simulink model "sistem_1"  (R2025b)
settings: Solver=VariableStepAuto  StartTime=0.0  StopTime=0.005  RelTol=1e-3
values from neighbouring files (symbols this model uses):
  c = 8e-08    [sistem_1.mat]
  K = 5.9098e-07    [sistem_1.mat]
  k_eq = 0.0291361239712    [sistem_1.mat]
  m_eq = 1.95689925e-12    [sistem_1.mat]
settings Model: Creator=RIZKI  LastModifiedBy=RIZKI

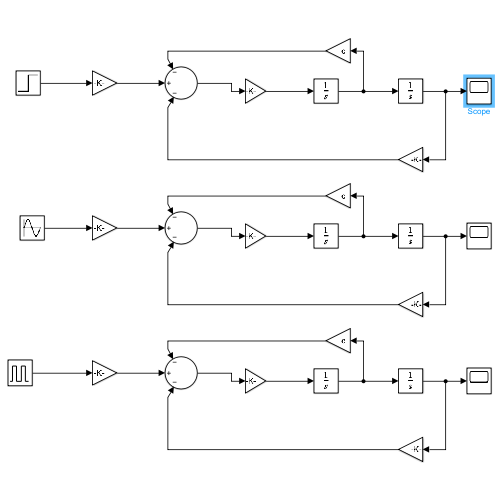
[thumbnail: Simulink's stored preview of the top-level diagram]
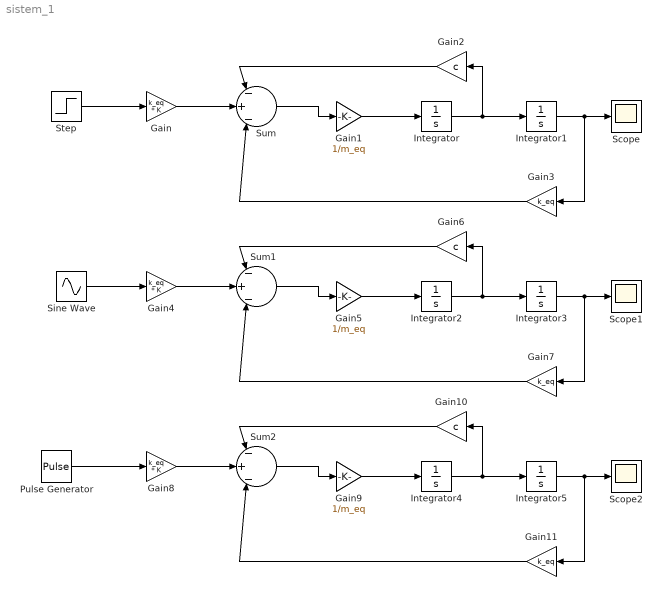
== system sistem_1 ==
  Gain : Gain  Gain=k_eq * K
  Gain1 : Gain  Gain=1/m_eq
  Gain10 : Gain  Gain=c
  Gain11 : Gain  Gain=k_eq
  Gain2 : Gain  Gain=c
  Gain3 : Gain  Gain=k_eq
  Gain4 : Gain  Gain=k_eq * K
  Gain5 : Gain  Gain=1/m_eq
  Gain6 : Gain  Gain=c
  Gain7 : Gain  Gain=k_eq
  Gain8 : Gain  Gain=k_eq * K
  Gain9 : Gain  Gain=1/m_eq
  Integrator{,1..5} (6 alike) : Integrator
  Pulse Generator : DiscretePulseGenerator  PulseType=Time based  Amplitude=20  Period=0.005
  Scope : Scope
      settings: ActiveDisplayYMinimum=9.91770131113692E-6  ActiveDisplayYMaximum=1.3466294857473047E-5
  Scope1 : Scope
      settings: ActiveDisplayYMinimum=-3.9428154732453781E-5  ActiveDisplayYMaximum=6.375855661608468E-5
  Scope2 : Scope
      settings: ActiveDisplayYMinimum=-6.032901409977137E-6  ActiveDisplayYMaximum=3.0264170830524335E-5  DataLoggingVariableName=ScopeData2
  Sine Wave : Sin  Amplitude=20  SampleTime=0
  Step : Step  Time=0  After=20  SampleTime=0
  Sum : Sum  Inputs=|-|+|-|
  Sum1 : Sum  Inputs=|-|+|-|
  Sum2 : Sum  Inputs=|-|+|-|
  wires:
  Step/1 -> Gain/1
  Sum/1 -> Gain1/1
  Gain1/1 -> Integrator/1
  Integrator/1 -> Gain2/1, Integrator1/1
  Integrator1/1 -> Gain3/1, Scope/1
  Gain3/1 -> Sum/3
  Gain/1 -> Sum/2
  Gain2/1 -> Sum/1
  Gain4/1 -> Sum1/2
  Integrator2/1 -> Gain6/1, Integrator3/1
  Gain7/1 -> Sum1/3
  Sum1/1 -> Gain5/1
  Gain6/1 -> Sum1/1
  Gain5/1 -> Integrator2/1
  Integrator3/1 -> Gain7/1, Scope1/1
  Sine Wave/1 -> Gain4/1
  Pulse Generator/1 -> Gain8/1
  Integrator5/1 -> Gain11/1, Scope2/1
  Gain10/1 -> Sum2/1
  Integrator4/1 -> Gain10/1, Integrator5/1
  Sum2/1 -> Gain9/1
  Gain11/1 -> Sum2/3
  Gain8/1 -> Sum2/2
  Gain9/1 -> Integrator4/1
